simulink model "test_s_function_design"  (R2014b)
settings: Solver=FixedStepDiscrete  StartTime=0.0  StopTime=300.0  FixedStep=0.1  RelTol=1e-3
InitFcn:
  | PockelsObject.clearPockels();
settings Model: Creator=kunalmenda  LastModifiedBy=kunalmenda

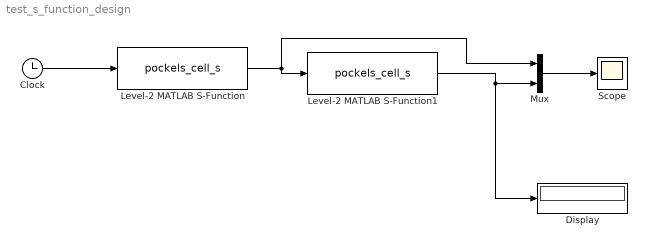
== system test_s_function_design ==
  Clock : Clock
  Display : Display
  Level-2 MATLAB S-Function : M-S-Function  FunctionName=pockels_cell_s  Parameters=P.PCTimings, P.ControlPowers  mask{PCTimings=[-1,1,38,40,103,105,168,170,220,274]*1e-9, ControlPowers=[0.5000, 1.0000,1.0000, 1.0000, 0.5000]}
      mask prompts: PCTimings "PC Timings"; ControlPowers "Control Powers"
      mask init:
      | P.PCTimings = PCTimings;
      | P.ControlPowers = ControlPowers;
  Level-2 MATLAB S-Function1 : M-S-Function  FunctionName=pockels_cell_s  Parameters=[-1,1,38,40,103,105,168,170,220,222,272,274]*1e-9, [0.5000, 1.0000,1.0000, 1.0000, 1.0000, 0.5000]
  Mux : Mux  Inputs=2
  Scope : Scope
  wires:
  Level-2 MATLAB S-Function/1 -> Level-2 MATLAB S-Function1/1, Mux/1
  Level-2 MATLAB S-Function1/1 -> Mux/2, Display/1
  Mux/1 -> Scope/1
  Clock/1 -> Level-2 MATLAB S-Function/1
